simulink model "fft32kpt_ssr16_fixed"  (R2024b)
settings: Solver=VariableStepAuto  StartTime=0.0  StopTime=sample_period*N*5  RelTol=1e-3
PreLoadFcn:
  | clk_freq = 570e6; % PL clock frequency
  | sample_period = 1/(570e6*16); % 570Msps*16parallel paths
  | N=32768; % fft point size
  | binw=(1/sample_period) / 2*N; % bin width
  | 
  | bin_freq = 2*pi*11*binw+pi*binw; % sin, cos freq centering per channel
  | 
  | % for transpose block
  | DATA_WIDTH=16;
  | SSR=16;
  | M=16;
  | N1=N/M;
  | MEM_STYLE=4; % MEM OPTIONS: 4 - ULTRA, 0 - AUTO, 1 - BRAM, 5 - MIXED
InitFcn:
  | clk_freq = 570e6; % PL clock frequency
  | sample_period = 1/(570e6*16); % 570Msps*16parallel paths
  | N=32768; % fft point size
  | binw=(1/sample_period) / 2*N; % bin width
  | 
  | bin_freq = 2*pi*11*binw+pi*binw; % sin, cos freq centering per channel
  | 
  | % for transpose block
  | DATA_WIDTH=16;
  | SSR=16;
  | M=16;
  | N1=N/M;
  | MEM_STYLE=4; % MEM OPTIONS: 4 - ULTRA, 0 - AUTO, 1 - BRAM, 5 - MIXED
undefined symbols (not defined in the file or in its folder): None, S, vsva2197, xcvc1902
libraries: aieBasic x47, hdlBasic x39, aieUtilities x16, aieDSP x16, hdlUtilities x16, matrix_library x16, hdlSSR x13, simulink x1, dspxfrm3 x1, vmcUtilities x1
(part 2 of 3)

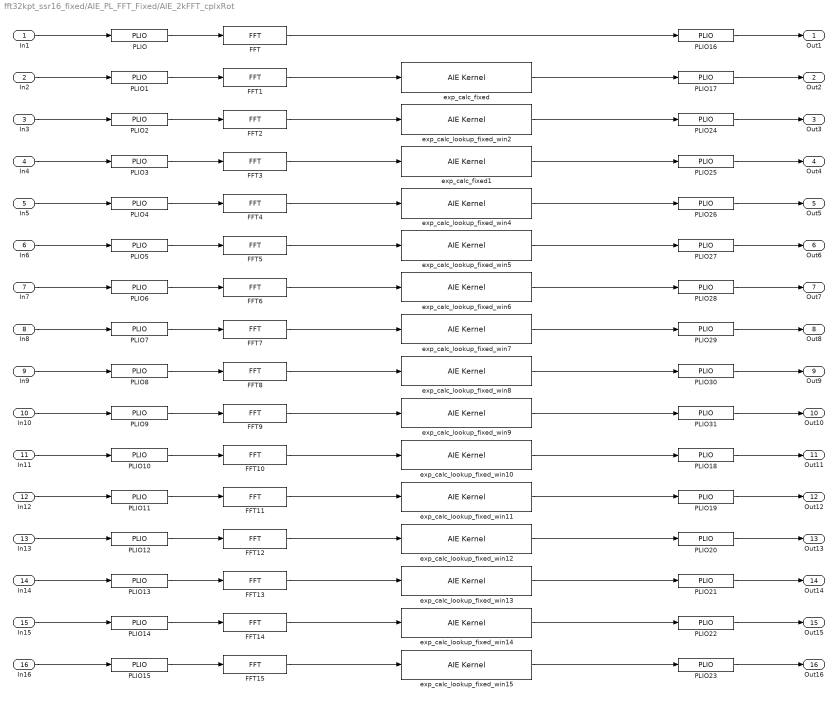
== system fft32kpt_ssr16_fixed/AIE_PL_FFT_Fixed/AIE_2kFFT_cplxRot ==
  In1 : Inport
  In2 : Inport  Port=2
  In3 : Inport  Port=3
  In4 : Inport  Port=4
  In5 : Inport  Port=5
  In6 : Inport  Port=6
  In7 : Inport  Port=7
  In8 : Inport  Port=8
  In9 : Inport  Port=9
  In10 : Inport  Port=10
  In11 : Inport  Port=11
  In12 : Inport  Port=12
  In13 : Inport  Port=13
  In14 : Inport  Port=14
  In15 : Inport  Port=15
  In16 : Inport  Port=16
  FFT{,1..15} (16 alike) : aieDSP/FFT  AIE_VARIANT=1  data_type=cint16  data_out_type=cint16  twiddle_type=cint16  point_size=2048  input_window_size=2048  shift_val=11  rnd_mode=Round symmetrical to infinity  sat_mode=0-None  ssr=1  twiddle_mode=0  use_ssr_widget_kernels=off  casc_length=1  transform_fft_nifft=1  TP_API=0  TP_DYN_PT_SIZE=0  blockJsonConstraints=[]  blockJsonConstraintsInternal=[]  spec=vmc_fft.json  SerializedMaskParamNames=[]  SerializedMaskParamValues=[]  SerializedMaskParamVisibilities=[]  block_type=FFT  SerializedMaskParamDataypes=uint|typename|typename|typename|uint|uint|uint|uint|uint|uint|uint|uint|uint|uint|uint|uint  SerializedMaskParamEnumStrArr=0|0|0|0|0|0|0|Round to positive infinity,Round to negative infinity,Round symmetrical to infinity,Round symmetrical to zero,Round convergent to even,Round convergent to odd|0-None,1-Asymmetric,3-Symmetric|0|0|0|0|0|0|0  SerializedMaskParamEnumValArr=0|0|0|0|0|0|0|2,3,4,5,6,7|0,1,3|0|0|0|0|0|0|0  SerializedMaskParamVectorArr=0|0|0|0|0|0|0|0|0|0|0|0|0|0|0|0  SerializedMaskParamKeys=AIE_VARIANT|TT_DATA|TT_OUT_DATA|TT_TWIDDLE|TP_POINT_SIZE|TP_WINDOW_VSIZE|TP_SHIFT|TP_RND|TP_SAT|TP_PARALLEL_POWER|TP_TWIDDLE_MODE|TP_USE_WIDGETS|TP_CASC_LEN|TP_FFT_NIFFT|TP_API|TP_DYN_PT_SIZE
  PLIO{,1..31} (32 alike) : aieBasic/PLIO  PlioWidth=64  PlioFreqSpec=on  PlioFreq=clk_freq/1e6  ColLocation=0  channel=0  blockJsonConstraints=[]  deprecateConstraints=0
  exp_calc_fixed : aieBasic/AIE Kernel  KernelAllAttrs=|  PortNames={'cb_input1'; 'cb_output1'}  PortSerializedTypes={'{Q2{R{Tadf::input_buffer{1{t{Scint16}}}}}}'; '{Q2{R{Tadf::output_buffer{1{t{Scint16}}}}}}'}  PortWindowSizes={2.048000000000000000e+03, 2.048000000000000000e+03}  PortWindowMargins={0.000000000000000000e+00, 0.000000000000000000e+00}  PortSynchronicities={'sync', 'sync'}  PortSignalSizes={0.000000000000000000e+00; 0.000000000000000000e+00}  FunctionTemplateSpecKind=implicit  FunctionTemplateParamNames={'PHASE_INDEX'}  FunctionTemplateParamKinds={'nontype'}  FunctionTemplateParamTypes={'unsigned int'}  FunctionTemplateParamValues={'1'}  FunctionIndex=1  FunctionTabVisible=on  FunctionTemplateParamsVisible=on  FunctionDeclTypeOptions=|  FunctionDecl=|  FunctionTemplateParams={ 'PHASE_INDEX', 'unsigned int', '1' }  FunctionTemplateParamsEnables={'off', 'off', 'on'}  PortAttrs={ 'input', 'cb_input1', 'adf::input_buffer< cint16 > & restrict', '2048', '0', 'sync', ''; 'output', 'cb_output1', 'adf::output_buffer< cint16 > & restrict', '2048', '', 'sync', '' }  PortAttrsEnables={'off', 'off', 'off', 'on', 'off', 'off', 'off';'off', 'off', 'off', 'on', 'off', 'off', 'off'}  SampleTime=-1  KernelHeaderFile=exp_calc_fixed.h  KernelFunction=exp_calc_fixed  KernelSourceFile=exp_calc_fixed.cc  KernelSearchPaths={}  PreProcOptions={}  blockJsonConstraints="{\"type\":\"constraint\",\"constraintType\":\"coreUtilization\",\"sid\":\"3274\",\"lhs\":{\"type\":\"runtimeRatio\",\"args\":{\"type\":\"kernel\",\"name\":\"fft32kpt_int_xpose_rrlto/AIE_2kFFT_cplxRot/exp_calc_lookup_fixed_win1\",\"sid\":\"3274\"}},\"rhs\":{\"type\":\"evaluable\",\"expr\":\"0.2\",\"value\":0.2},\"equality\":true}"
      KernelAllAttrs=|
      | s[12;12;9;9;19;14;21;23;21;23;24;21;15;17;12;24;26;26;26;27;28;9;21;23;23;23;24;25;14;19;19;29]@FunctionNameDeclFileNamePortNamesPortTypesPortSerializedTypesPortDirectionsPortWindowSizeEnablesPortWindowMarginEnablesPortBufferSizeEnablesPortBufferMarginEnablesPortSynchronicityEnablesPortSignalSizeEnablesPortBufferSizesPortBufferMarginsFunctionDeclFunctionTemplateSpecKindFunctionTemplateParamNamesFunctionTemplateParamKindsFunctionTemplateParamTypesFunctionTemplateParamValuesFunctionTemplateParamEnablesClassDeclClassTemplateSpecKindClassTemplateParamNamesClassTemplateParamKindsClassTemplateParamTypesClassTemplateParamValuesClassTemplateParamEnablesClassCtorDeclsClassCtorParamNamesClassCtorParamTypesClassCtorParamSerializedTypes[1 1]@C[32 1]@t14@exp_calc_fixedt22@../../exp_calc_fixed.hC[2 1]@t9@cb_input1t10@cb_output1C[2 1]@t38@adf::input_buffer< cint16 > & restrictt39@adf::output_buffer< cint16 > & restrictC[2 1]@t42@{Q2{R{Tadf::input_buffer{1{t{Scint16}}}}}}t43@{Q2{R{Tadf::output_buffer{1{t{Scint16}}}}}}C[2 1]@t5@inputt6@outputC[2 1]@l1@l1@C[2 1]@l1@l0@C[2 1]@l1@l1@C[2 1]@l0@l0@C[2 1]@l1@l1@C[2 1]@l0@l0@C[2 1]@nnC[2 1]@nnt160@template < unsigned int PHASE_INDEX > 
      | void exp_calc_fixed(adf::input_buffer< cint16 > & restrict cb_input1, adf::output_buffer< cint16 > & restrict cb_output1)t8@implicitC[1 1]@t11@PHASE_INDEXC[1 1]@t7@nontypeC[1 1]@t12@unsigned intC[1 1]@nC[1 1]@l1@nne[0 1]@e[0 1]@e[0 1]@e[0 1]@e[0 1]@e[0 1]@e[0 1]@e[0 1]@e[0 1]@
      FunctionDeclTypeOptions=|
      | C[1 1]@t162@template < unsigned int PHASE_INDEX > 
      | void exp_calc_fixed(adf::input_buffer< cint16 > && restrict cb_input1, adf::output_buffer< cint16 > && restrict cb_output1)
      FunctionDecl=|
      | template < unsigned int PHASE_INDEX > 
      | void exp_calc_fixed(adf::input_buffer< cint16 > && restrict cb_input1, adf::output_buffer< cint16 > && restrict cb_output1)
  exp_calc_fixed1 : aieBasic/AIE Kernel  KernelAllAttrs=|  PortNames={'cb_input1'; 'cb_output1'}  PortSerializedTypes={'{Q2{R{Tadf::input_buffer{1{t{Scint16}}}}}}'; '{Q2{R{Tadf::output_buffer{1{t{Scint16}}}}}}'}  PortWindowSizes={2.048000000000000000e+03, 2.048000000000000000e+03}  PortWindowMargins={0.000000000000000000e+00, 0.000000000000000000e+00}  PortSynchronicities={'sync', 'sync'}  PortSignalSizes={0.000000000000000000e+00; 0.000000000000000000e+00}  FunctionTemplateSpecKind=implicit  FunctionTemplateParamNames={'PHASE_INDEX'}  FunctionTemplateParamKinds={'nontype'}  FunctionTemplateParamTypes={'unsigned int'}  FunctionTemplateParamValues={'3'}  FunctionIndex=1  FunctionTabVisible=on  FunctionTemplateParamsVisible=on  FunctionDeclTypeOptions=|  FunctionDecl=|  FunctionTemplateParams={ 'PHASE_INDEX', 'unsigned int', '3' }  FunctionTemplateParamsEnables={'off', 'off', 'on'}  PortAttrs={ 'input', 'cb_input1', 'adf::input_buffer< cint16 > & restrict', '2048', '0', 'sync', ''; 'output', 'cb_output1', 'adf::output_buffer< cint16 > & restrict', '2048', '', 'sync', '' }  PortAttrsEnables={'off', 'off', 'off', 'on', 'off', 'off', 'off';'off', 'off', 'off', 'on', 'off', 'off', 'off'}  SampleTime=-1  KernelHeaderFile=exp_calc_fixed.h  KernelFunction=exp_calc_fixed  KernelSourceFile=exp_calc_fixed.cc  KernelSearchPaths={}  PreProcOptions={}  blockJsonConstraints="{\"type\":\"constraint\",\"constraintType\":\"coreUtilization\",\"sid\":\"3282\",\"lhs\":{\"type\":\"runtimeRatio\",\"args\":{\"type\":\"kernel\",\"name\":\"fft32kpt_int_xpose/AIE_2kFFT_cplxRot/exp_calc_lookup_fixed_win3\",\"sid\":\"3282\"}},\"rhs\":{\"type\":\"evaluable\",\"expr\":\"0.2\",\"value\":0.2},\"equality\":true}"
      KernelAllAttrs=|
      | s[12;12;9;9;19;14;21;23;21;23;24;21;15;17;12;24;26;26;26;27;28;9;21;23;23;23;24;25;14;19;19;29]@FunctionNameDeclFileNamePortNamesPortTypesPortSerializedTypesPortDirectionsPortWindowSizeEnablesPortWindowMarginEnablesPortBufferSizeEnablesPortBufferMarginEnablesPortSynchronicityEnablesPortSignalSizeEnablesPortBufferSizesPortBufferMarginsFunctionDeclFunctionTemplateSpecKindFunctionTemplateParamNamesFunctionTemplateParamKindsFunctionTemplateParamTypesFunctionTemplateParamValuesFunctionTemplateParamEnablesClassDeclClassTemplateSpecKindClassTemplateParamNamesClassTemplateParamKindsClassTemplateParamTypesClassTemplateParamValuesClassTemplateParamEnablesClassCtorDeclsClassCtorParamNamesClassCtorParamTypesClassCtorParamSerializedTypes[1 1]@C[32 1]@t14@exp_calc_fixedt22@../../exp_calc_fixed.hC[2 1]@t9@cb_input1t10@cb_output1C[2 1]@t38@adf::input_buffer< cint16 > & restrictt39@adf::output_buffer< cint16 > & restrictC[2 1]@t42@{Q2{R{Tadf::input_buffer{1{t{Scint16}}}}}}t43@{Q2{R{Tadf::output_buffer{1{t{Scint16}}}}}}C[2 1]@t5@inputt6@outputC[2 1]@l1@l1@C[2 1]@l1@l0@C[2 1]@l1@l1@C[2 1]@l0@l0@C[2 1]@l1@l1@C[2 1]@l0@l0@C[2 1]@nnC[2 1]@nnt160@template < unsigned int PHASE_INDEX > 
      | void exp_calc_fixed(adf::input_buffer< cint16 > & restrict cb_input1, adf::output_buffer< cint16 > & restrict cb_output1)t8@implicitC[1 1]@t11@PHASE_INDEXC[1 1]@t7@nontypeC[1 1]@t12@unsigned intC[1 1]@nC[1 1]@l1@nne[0 1]@e[0 1]@e[0 1]@e[0 1]@e[0 1]@e[0 1]@e[0 1]@e[0 1]@e[0 1]@
      FunctionDeclTypeOptions=|
      | C[1 1]@t162@template < unsigned int PHASE_INDEX > 
      | void exp_calc_fixed(adf::input_buffer< cint16 > && restrict cb_input1, adf::output_buffer< cint16 > && restrict cb_output1)
      FunctionDecl=|
      | template < unsigned int PHASE_INDEX > 
      | void exp_calc_fixed(adf::input_buffer< cint16 > && restrict cb_input1, adf::output_buffer< cint16 > && restrict cb_output1)
  exp_calc_lookup_fixed_win10 : aieBasic/AIE Kernel  KernelAllAttrs=|  PortNames={'cb_input1'; 'cb_output1'}  PortSerializedTypes={'{Q2{R{Tadf::input_buffer{1{t{Scint16}}}}}}'; '{Q2{R{Tadf::output_buffer{1{t{Scint16}}}}}}'}  PortWindowSizes={2.048000000000000000e+03, 2.048000000000000000e+03}  PortWindowMargins={0.000000000000000000e+00, 0.000000000000000000e+00}  PortSynchronicities={'sync', 'sync'}  PortSignalSizes={0.000000000000000000e+00; 0.000000000000000000e+00}  FunctionTemplateSpecKind=implicit  FunctionTemplateParamNames={'PHASE_INDEX'}  FunctionTemplateParamKinds={'nontype'}  FunctionTemplateParamTypes={'unsigned int'}  FunctionTemplateParamValues={'10'}  FunctionIndex=1  FunctionTabVisible=on  FunctionTemplateParamsVisible=on  FunctionDeclTypeOptions=|  FunctionDecl=|  FunctionTemplateParams={ 'PHASE_INDEX', 'unsigned int', '10' }  FunctionTemplateParamsEnables={'off', 'off', 'on'}  PortAttrs={ 'input', 'cb_input1', 'adf::input_buffer< cint16 > & restrict', '2048', '0', 'sync', ''; 'output', 'cb_output1', 'adf::output_buffer< cint16 > & restrict', '2048', '', 'sync', '' }  PortAttrsEnables={'off', 'off', 'off', 'on', 'off', 'off', 'off';'off', 'off', 'off', 'on', 'off', 'off', 'off'}  SampleTime=-1  KernelHeaderFile=exp_calc_fixed.h  KernelFunction=exp_calc_fixed  KernelSourceFile=exp_calc_fixed.cc  KernelSearchPaths={}  PreProcOptions={}  blockJsonConstraints="{\"type\":\"constraint\",\"constraintType\":\"coreUtilization\",\"sid\":\"3275\",\"lhs\":{\"type\":\"runtimeRatio\",\"args\":{\"type\":\"kernel\",\"name\":\"fft32kpt_int_xpose_rrlto/AIE_2kFFT_cplxRot/exp_calc_lookup_fixed_win10\",\"sid\":\"3275\"}},\"rhs\":{\"type\":\"evaluable\",\"expr\":\"0.2\",\"value\":0.2},\"equality\":true}"
      KernelAllAttrs=|
      | s[12;12;9;9;19;14;21;23;21;23;24;21;15;17;12;24;26;26;26;27;28;9;21;23;23;23;24;25;14;19;19;29]@FunctionNameDeclFileNamePortNamesPortTypesPortSerializedTypesPortDirectionsPortWindowSizeEnablesPortWindowMarginEnablesPortBufferSizeEnablesPortBufferMarginEnablesPortSynchronicityEnablesPortSignalSizeEnablesPortBufferSizesPortBufferMarginsFunctionDeclFunctionTemplateSpecKindFunctionTemplateParamNamesFunctionTemplateParamKindsFunctionTemplateParamTypesFunctionTemplateParamValuesFunctionTemplateParamEnablesClassDeclClassTemplateSpecKindClassTemplateParamNamesClassTemplateParamKindsClassTemplateParamTypesClassTemplateParamValuesClassTemplateParamEnablesClassCtorDeclsClassCtorParamNamesClassCtorParamTypesClassCtorParamSerializedTypes[1 1]@C[32 1]@t14@exp_calc_fixedt22@../../exp_calc_fixed.hC[2 1]@t9@cb_input1t10@cb_output1C[2 1]@t38@adf::input_buffer< cint16 > & restrictt39@adf::output_buffer< cint16 > & restrictC[2 1]@t42@{Q2{R{Tadf::input_buffer{1{t{Scint16}}}}}}t43@{Q2{R{Tadf::output_buffer{1{t{Scint16}}}}}}C[2 1]@t5@inputt6@outputC[2 1]@l1@l1@C[2 1]@l1@l0@C[2 1]@l1@l1@C[2 1]@l0@l0@C[2 1]@l1@l1@C[2 1]@l0@l0@C[2 1]@nnC[2 1]@nnt160@template < unsigned int PHASE_INDEX > 
      | void exp_calc_fixed(adf::input_buffer< cint16 > & restrict cb_input1, adf::output_buffer< cint16 > & restrict cb_output1)t8@implicitC[1 1]@t11@PHASE_INDEXC[1 1]@t7@nontypeC[1 1]@t12@unsigned intC[1 1]@nC[1 1]@l1@nne[0 1]@e[0 1]@e[0 1]@e[0 1]@e[0 1]@e[0 1]@e[0 1]@e[0 1]@e[0 1]@
      FunctionDeclTypeOptions=|
      | C[1 1]@t162@template < unsigned int PHASE_INDEX > 
      | void exp_calc_fixed(adf::input_buffer< cint16 > && restrict cb_input1, adf::output_buffer< cint16 > && restrict cb_output1)
      FunctionDecl=|
      | template < unsigned int PHASE_INDEX > 
      | void exp_calc_fixed(adf::input_buffer< cint16 > && restrict cb_input1, adf::output_buffer< cint16 > && restrict cb_output1)
  exp_calc_lookup_fixed_win11 : aieBasic/AIE Kernel  KernelAllAttrs=|  PortNames={'cb_input1'; 'cb_output1'}  PortSerializedTypes={'{Q2{R{Tadf::input_buffer{1{t{Scint16}}}}}}'; '{Q2{R{Tadf::output_buffer{1{t{Scint16}}}}}}'}  PortWindowSizes={2.048000000000000000e+03, 2.048000000000000000e+03}  PortWindowMargins={0.000000000000000000e+00, 0.000000000000000000e+00}  PortSynchronicities={'sync', 'sync'}  PortSignalSizes={0.000000000000000000e+00; 0.000000000000000000e+00}  FunctionTemplateSpecKind=implicit  FunctionTemplateParamNames={'PHASE_INDEX'}  FunctionTemplateParamKinds={'nontype'}  FunctionTemplateParamTypes={'unsigned int'}  FunctionTemplateParamValues={'11'}  FunctionIndex=1  FunctionTabVisible=on  FunctionTemplateParamsVisible=on  FunctionDeclTypeOptions=|  FunctionDecl=|  FunctionTemplateParams={ 'PHASE_INDEX', 'unsigned int', '11' }  FunctionTemplateParamsEnables={'off', 'off', 'on'}  PortAttrs={ 'input', 'cb_input1', 'adf::input_buffer< cint16 > & restrict', '2048', '0', 'sync', ''; 'output', 'cb_output1', 'adf::output_buffer< cint16 > & restrict', '2048', '', 'sync', '' }  PortAttrsEnables={'off', 'off', 'off', 'on', 'off', 'off', 'off';'off', 'off', 'off', 'on', 'off', 'off', 'off'}  SampleTime=-1  KernelHeaderFile=exp_calc_fixed.h  KernelFunction=exp_calc_fixed  KernelSourceFile=exp_calc_fixed.cc  KernelSearchPaths={}  PreProcOptions={}  blockJsonConstraints="{\"type\":\"constraint\",\"constraintType\":\"coreUtilization\",\"sid\":\"3276\",\"lhs\":{\"type\":\"runtimeRatio\",\"args\":{\"type\":\"kernel\",\"name\":\"fft32kpt_int_xpose/AIE_2kFFT_cplxRot/exp_calc_lookup_fixed_win11\",\"sid\":\"3276\"}},\"rhs\":{\"type\":\"evaluable\",\"expr\":\"0.2\",\"value\":0.2},\"equality\":true}"
      KernelAllAttrs=|
      | s[12;12;9;9;19;14;21;23;21;23;24;21;15;17;12;24;26;26;26;27;28;9;21;23;23;23;24;25;14;19;19;29]@FunctionNameDeclFileNamePortNamesPortTypesPortSerializedTypesPortDirectionsPortWindowSizeEnablesPortWindowMarginEnablesPortBufferSizeEnablesPortBufferMarginEnablesPortSynchronicityEnablesPortSignalSizeEnablesPortBufferSizesPortBufferMarginsFunctionDeclFunctionTemplateSpecKindFunctionTemplateParamNamesFunctionTemplateParamKindsFunctionTemplateParamTypesFunctionTemplateParamValuesFunctionTemplateParamEnablesClassDeclClassTemplateSpecKindClassTemplateParamNamesClassTemplateParamKindsClassTemplateParamTypesClassTemplateParamValuesClassTemplateParamEnablesClassCtorDeclsClassCtorParamNamesClassCtorParamTypesClassCtorParamSerializedTypes[1 1]@C[32 1]@t14@exp_calc_fixedt22@../../exp_calc_fixed.hC[2 1]@t9@cb_input1t10@cb_output1C[2 1]@t38@adf::input_buffer< cint16 > & restrictt39@adf::output_buffer< cint16 > & restrictC[2 1]@t42@{Q2{R{Tadf::input_buffer{1{t{Scint16}}}}}}t43@{Q2{R{Tadf::output_buffer{1{t{Scint16}}}}}}C[2 1]@t5@inputt6@outputC[2 1]@l1@l1@C[2 1]@l1@l0@C[2 1]@l1@l1@C[2 1]@l0@l0@C[2 1]@l1@l1@C[2 1]@l0@l0@C[2 1]@nnC[2 1]@nnt160@template < unsigned int PHASE_INDEX > 
      | void exp_calc_fixed(adf::input_buffer< cint16 > & restrict cb_input1, adf::output_buffer< cint16 > & restrict cb_output1)t8@implicitC[1 1]@t11@PHASE_INDEXC[1 1]@t7@nontypeC[1 1]@t12@unsigned intC[1 1]@nC[1 1]@l1@nne[0 1]@e[0 1]@e[0 1]@e[0 1]@e[0 1]@e[0 1]@e[0 1]@e[0 1]@e[0 1]@
      FunctionDeclTypeOptions=|
      | C[1 1]@t162@template < unsigned int PHASE_INDEX > 
      | void exp_calc_fixed(adf::input_buffer< cint16 > && restrict cb_input1, adf::output_buffer< cint16 > && restrict cb_output1)
      FunctionDecl=|
      | template < unsigned int PHASE_INDEX > 
      | void exp_calc_fixed(adf::input_buffer< cint16 > && restrict cb_input1, adf::output_buffer< cint16 > && restrict cb_output1)
  exp_calc_lookup_fixed_win12 : aieBasic/AIE Kernel  KernelAllAttrs=|  PortNames={'cb_input1'; 'cb_output1'}  PortSerializedTypes={'{Q2{R{Tadf::input_buffer{1{t{Scint16}}}}}}'; '{Q2{R{Tadf::output_buffer{1{t{Scint16}}}}}}'}  PortWindowSizes={2.048000000000000000e+03, 2.048000000000000000e+03}  PortWindowMargins={0.000000000000000000e+00, 0.000000000000000000e+00}  PortSynchronicities={'sync', 'sync'}  PortSignalSizes={0.000000000000000000e+00; 0.000000000000000000e+00}  FunctionTemplateSpecKind=implicit  FunctionTemplateParamNames={'PHASE_INDEX'}  FunctionTemplateParamKinds={'nontype'}  FunctionTemplateParamTypes={'unsigned int'}  FunctionTemplateParamValues={'12'}  FunctionIndex=1  FunctionTabVisible=on  FunctionTemplateParamsVisible=on  FunctionDeclTypeOptions=|  FunctionDecl=|  FunctionTemplateParams={ 'PHASE_INDEX', 'unsigned int', '12' }  FunctionTemplateParamsEnables={'off', 'off', 'on'}  PortAttrs={ 'input', 'cb_input1', 'adf::input_buffer< cint16 > & restrict', '2048', '0', 'sync', ''; 'output', 'cb_output1', 'adf::output_buffer< cint16 > & restrict', '2048', '', 'sync', '' }  PortAttrsEnables={'off', 'off', 'off', 'on', 'off', 'off', 'off';'off', 'off', 'off', 'on', 'off', 'off', 'off'}  SampleTime=-1  KernelHeaderFile=exp_calc_fixed.h  KernelFunction=exp_calc_fixed  KernelSourceFile=exp_calc_fixed.cc  KernelSearchPaths={}  PreProcOptions={}  blockJsonConstraints="{\"type\":\"constraint\",\"constraintType\":\"coreUtilization\",\"sid\":\"3277\",\"lhs\":{\"type\":\"runtimeRatio\",\"args\":{\"type\":\"kernel\",\"name\":\"fft32kpt_int_xpose/AIE_2kFFT_cplxRot/exp_calc_lookup_fixed_win12\",\"sid\":\"3277\"}},\"rhs\":{\"type\":\"evaluable\",\"expr\":\"0.2\",\"value\":0.2},\"equality\":true}"
      KernelAllAttrs=|
      | s[12;12;9;9;19;14;21;23;21;23;24;21;15;17;12;24;26;26;26;27;28;9;21;23;23;23;24;25;14;19;19;29]@FunctionNameDeclFileNamePortNamesPortTypesPortSerializedTypesPortDirectionsPortWindowSizeEnablesPortWindowMarginEnablesPortBufferSizeEnablesPortBufferMarginEnablesPortSynchronicityEnablesPortSignalSizeEnablesPortBufferSizesPortBufferMarginsFunctionDeclFunctionTemplateSpecKindFunctionTemplateParamNamesFunctionTemplateParamKindsFunctionTemplateParamTypesFunctionTemplateParamValuesFunctionTemplateParamEnablesClassDeclClassTemplateSpecKindClassTemplateParamNamesClassTemplateParamKindsClassTemplateParamTypesClassTemplateParamValuesClassTemplateParamEnablesClassCtorDeclsClassCtorParamNamesClassCtorParamTypesClassCtorParamSerializedTypes[1 1]@C[32 1]@t14@exp_calc_fixedt22@../../exp_calc_fixed.hC[2 1]@t9@cb_input1t10@cb_output1C[2 1]@t38@adf::input_buffer< cint16 > & restrictt39@adf::output_buffer< cint16 > & restrictC[2 1]@t42@{Q2{R{Tadf::input_buffer{1{t{Scint16}}}}}}t43@{Q2{R{Tadf::output_buffer{1{t{Scint16}}}}}}C[2 1]@t5@inputt6@outputC[2 1]@l1@l1@C[2 1]@l1@l0@C[2 1]@l1@l1@C[2 1]@l0@l0@C[2 1]@l1@l1@C[2 1]@l0@l0@C[2 1]@nnC[2 1]@nnt160@template < unsigned int PHASE_INDEX > 
      | void exp_calc_fixed(adf::input_buffer< cint16 > & restrict cb_input1, adf::output_buffer< cint16 > & restrict cb_output1)t8@implicitC[1 1]@t11@PHASE_INDEXC[1 1]@t7@nontypeC[1 1]@t12@unsigned intC[1 1]@nC[1 1]@l1@nne[0 1]@e[0 1]@e[0 1]@e[0 1]@e[0 1]@e[0 1]@e[0 1]@e[0 1]@e[0 1]@
      FunctionDeclTypeOptions=|
      | C[1 1]@t162@template < unsigned int PHASE_INDEX > 
      | void exp_calc_fixed(adf::input_buffer< cint16 > && restrict cb_input1, adf::output_buffer< cint16 > && restrict cb_output1)
      FunctionDecl=|
      | template < unsigned int PHASE_INDEX > 
      | void exp_calc_fixed(adf::input_buffer< cint16 > && restrict cb_input1, adf::output_buffer< cint16 > && restrict cb_output1)
  exp_calc_lookup_fixed_win13 : aieBasic/AIE Kernel  KernelAllAttrs=|  PortNames={'cb_input1'; 'cb_output1'}  PortSerializedTypes={'{Q2{R{Tadf::input_buffer{1{t{Scint16}}}}}}'; '{Q2{R{Tadf::output_buffer{1{t{Scint16}}}}}}'}  PortWindowSizes={2.048000000000000000e+03, 2.048000000000000000e+03}  PortWindowMargins={0.000000000000000000e+00, 0.000000000000000000e+00}  PortSynchronicities={'sync', 'sync'}  PortSignalSizes={0.000000000000000000e+00; 0.000000000000000000e+00}  FunctionTemplateSpecKind=implicit  FunctionTemplateParamNames={'PHASE_INDEX'}  FunctionTemplateParamKinds={'nontype'}  FunctionTemplateParamTypes={'unsigned int'}  FunctionTemplateParamValues={'13'}  FunctionIndex=1  FunctionTabVisible=on  FunctionTemplateParamsVisible=on  FunctionDeclTypeOptions=|  FunctionDecl=|  FunctionTemplateParams={ 'PHASE_INDEX', 'unsigned int', '13' }  FunctionTemplateParamsEnables={'off', 'off', 'on'}  PortAttrs={ 'input', 'cb_input1', 'adf::input_buffer< cint16 > & restrict', '2048', '0', 'sync', ''; 'output', 'cb_output1', 'adf::output_buffer< cint16 > & restrict', '2048', '', 'sync', '' }  PortAttrsEnables={'off', 'off', 'off', 'on', 'off', 'off', 'off';'off', 'off', 'off', 'on', 'off', 'off', 'off'}  SampleTime=-1  KernelHeaderFile=exp_calc_fixed.h  KernelFunction=exp_calc_fixed  KernelSourceFile=exp_calc_fixed.cc  KernelSearchPaths={}  PreProcOptions={}  blockJsonConstraints="{\"type\":\"constraint\",\"constraintType\":\"coreUtilization\",\"sid\":\"3278\",\"lhs\":{\"type\":\"runtimeRatio\",\"args\":{\"type\":\"kernel\",\"name\":\"fft32kpt_int_xpose/AIE_2kFFT_cplxRot/exp_calc_lookup_fixed_win13\",\"sid\":\"3278\"}},\"rhs\":{\"type\":\"evaluable\",\"expr\":\"0.2\",\"value\":0.2},\"equality\":true}"
      KernelAllAttrs=|
      | s[12;12;9;9;19;14;21;23;21;23;24;21;15;17;12;24;26;26;26;27;28;9;21;23;23;23;24;25;14;19;19;29]@FunctionNameDeclFileNamePortNamesPortTypesPortSerializedTypesPortDirectionsPortWindowSizeEnablesPortWindowMarginEnablesPortBufferSizeEnablesPortBufferMarginEnablesPortSynchronicityEnablesPortSignalSizeEnablesPortBufferSizesPortBufferMarginsFunctionDeclFunctionTemplateSpecKindFunctionTemplateParamNamesFunctionTemplateParamKindsFunctionTemplateParamTypesFunctionTemplateParamValuesFunctionTemplateParamEnablesClassDeclClassTemplateSpecKindClassTemplateParamNamesClassTemplateParamKindsClassTemplateParamTypesClassTemplateParamValuesClassTemplateParamEnablesClassCtorDeclsClassCtorParamNamesClassCtorParamTypesClassCtorParamSerializedTypes[1 1]@C[32 1]@t14@exp_calc_fixedt22@../../exp_calc_fixed.hC[2 1]@t9@cb_input1t10@cb_output1C[2 1]@t38@adf::input_buffer< cint16 > & restrictt39@adf::output_buffer< cint16 > & restrictC[2 1]@t42@{Q2{R{Tadf::input_buffer{1{t{Scint16}}}}}}t43@{Q2{R{Tadf::output_buffer{1{t{Scint16}}}}}}C[2 1]@t5@inputt6@outputC[2 1]@l1@l1@C[2 1]@l1@l0@C[2 1]@l1@l1@C[2 1]@l0@l0@C[2 1]@l1@l1@C[2 1]@l0@l0@C[2 1]@nnC[2 1]@nnt160@template < unsigned int PHASE_INDEX > 
      | void exp_calc_fixed(adf::input_buffer< cint16 > & restrict cb_input1, adf::output_buffer< cint16 > & restrict cb_output1)t8@implicitC[1 1]@t11@PHASE_INDEXC[1 1]@t7@nontypeC[1 1]@t12@unsigned intC[1 1]@nC[1 1]@l1@nne[0 1]@e[0 1]@e[0 1]@e[0 1]@e[0 1]@e[0 1]@e[0 1]@e[0 1]@e[0 1]@
      FunctionDeclTypeOptions=|
      | C[1 1]@t162@template < unsigned int PHASE_INDEX > 
      | void exp_calc_fixed(adf::input_buffer< cint16 > && restrict cb_input1, adf::output_buffer< cint16 > && restrict cb_output1)
      FunctionDecl=|
      | template < unsigned int PHASE_INDEX > 
      | void exp_calc_fixed(adf::input_buffer< cint16 > && restrict cb_input1, adf::output_buffer< cint16 > && restrict cb_output1)
  exp_calc_lookup_fixed_win14 : aieBasic/AIE Kernel  KernelAllAttrs=|  PortNames={'cb_input1'; 'cb_output1'}  PortSerializedTypes={'{Q2{R{Tadf::input_buffer{1{t{Scint16}}}}}}'; '{Q2{R{Tadf::output_buffer{1{t{Scint16}}}}}}'}  PortWindowSizes={2.048000000000000000e+03, 2.048000000000000000e+03}  PortWindowMargins={0.000000000000000000e+00, 0.000000000000000000e+00}  PortSynchronicities={'sync', 'sync'}  PortSignalSizes={0.000000000000000000e+00; 0.000000000000000000e+00}  FunctionTemplateSpecKind=implicit  FunctionTemplateParamNames={'PHASE_INDEX'}  FunctionTemplateParamKinds={'nontype'}  FunctionTemplateParamTypes={'unsigned int'}  FunctionTemplateParamValues={'14'}  FunctionIndex=1  FunctionTabVisible=on  FunctionTemplateParamsVisible=on  FunctionDeclTypeOptions=|  FunctionDecl=|  FunctionTemplateParams={ 'PHASE_INDEX', 'unsigned int', '14' }  FunctionTemplateParamsEnables={'off', 'off', 'on'}  PortAttrs={ 'input', 'cb_input1', 'adf::input_buffer< cint16 > & restrict', '2048', '0', 'sync', ''; 'output', 'cb_output1', 'adf::output_buffer< cint16 > & restrict', '2048', '', 'sync', '' }  PortAttrsEnables={'off', 'off', 'off', 'on', 'off', 'off', 'off';'off', 'off', 'off', 'on', 'off', 'off', 'off'}  SampleTime=-1  KernelHeaderFile=exp_calc_fixed.h  KernelFunction=exp_calc_fixed  KernelSourceFile=exp_calc_fixed.cc  KernelSearchPaths={}  PreProcOptions={}  blockJsonConstraints="{\"type\":\"constraint\",\"constraintType\":\"coreUtilization\",\"sid\":\"3279\",\"lhs\":{\"type\":\"runtimeRatio\",\"args\":{\"type\":\"kernel\",\"name\":\"fft32kpt_int_xpose/AIE_2kFFT_cplxRot/exp_calc_lookup_fixed_win14\",\"sid\":\"3279\"}},\"rhs\":{\"type\":\"evaluable\",\"expr\":\"0.2\",\"value\":0.2},\"equality\":true}"
      KernelAllAttrs=|
      | s[12;12;9;9;19;14;21;23;21;23;24;21;15;17;12;24;26;26;26;27;28;9;21;23;23;23;24;25;14;19;19;29]@FunctionNameDeclFileNamePortNamesPortTypesPortSerializedTypesPortDirectionsPortWindowSizeEnablesPortWindowMarginEnablesPortBufferSizeEnablesPortBufferMarginEnablesPortSynchronicityEnablesPortSignalSizeEnablesPortBufferSizesPortBufferMarginsFunctionDeclFunctionTemplateSpecKindFunctionTemplateParamNamesFunctionTemplateParamKindsFunctionTemplateParamTypesFunctionTemplateParamValuesFunctionTemplateParamEnablesClassDeclClassTemplateSpecKindClassTemplateParamNamesClassTemplateParamKindsClassTemplateParamTypesClassTemplateParamValuesClassTemplateParamEnablesClassCtorDeclsClassCtorParamNamesClassCtorParamTypesClassCtorParamSerializedTypes[1 1]@C[32 1]@t14@exp_calc_fixedt22@../../exp_calc_fixed.hC[2 1]@t9@cb_input1t10@cb_output1C[2 1]@t38@adf::input_buffer< cint16 > & restrictt39@adf::output_buffer< cint16 > & restrictC[2 1]@t42@{Q2{R{Tadf::input_buffer{1{t{Scint16}}}}}}t43@{Q2{R{Tadf::output_buffer{1{t{Scint16}}}}}}C[2 1]@t5@inputt6@outputC[2 1]@l1@l1@C[2 1]@l1@l0@C[2 1]@l1@l1@C[2 1]@l0@l0@C[2 1]@l1@l1@C[2 1]@l0@l0@C[2 1]@nnC[2 1]@nnt160@template < unsigned int PHASE_INDEX > 
      | void exp_calc_fixed(adf::input_buffer< cint16 > & restrict cb_input1, adf::output_buffer< cint16 > & restrict cb_output1)t8@implicitC[1 1]@t11@PHASE_INDEXC[1 1]@t7@nontypeC[1 1]@t12@unsigned intC[1 1]@nC[1 1]@l1@nne[0 1]@e[0 1]@e[0 1]@e[0 1]@e[0 1]@e[0 1]@e[0 1]@e[0 1]@e[0 1]@
      FunctionDeclTypeOptions=|
      | C[1 1]@t162@template < unsigned int PHASE_INDEX > 
      | void exp_calc_fixed(adf::input_buffer< cint16 > && restrict cb_input1, adf::output_buffer< cint16 > && restrict cb_output1)
      FunctionDecl=|
      | template < unsigned int PHASE_INDEX > 
      | void exp_calc_fixed(adf::input_buffer< cint16 > && restrict cb_input1, adf::output_buffer< cint16 > && restrict cb_output1)
  exp_calc_lookup_fixed_win15 : aieBasic/AIE Kernel  KernelAllAttrs=|  PortNames={'cb_input1'; 'cb_output1'}  PortSerializedTypes={'{Q2{R{Tadf::input_buffer{1{t{Scint16}}}}}}'; '{Q2{R{Tadf::output_buffer{1{t{Scint16}}}}}}'}  PortWindowSizes={2.048000000000000000e+03, 2.048000000000000000e+03}  PortWindowMargins={0.000000000000000000e+00, 0.000000000000000000e+00}  PortSynchronicities={'sync', 'sync'}  PortSignalSizes={0.000000000000000000e+00; 0.000000000000000000e+00}  FunctionTemplateSpecKind=implicit  FunctionTemplateParamNames={'PHASE_INDEX'}  FunctionTemplateParamKinds={'nontype'}  FunctionTemplateParamTypes={'unsigned int'}  FunctionTemplateParamValues={'15'}  FunctionIndex=1  FunctionTabVisible=on  FunctionTemplateParamsVisible=on  FunctionDeclTypeOptions=|  FunctionDecl=|  FunctionTemplateParams={ 'PHASE_INDEX', 'unsigned int', '15' }  FunctionTemplateParamsEnables={'off', 'off', 'on'}  PortAttrs={ 'input', 'cb_input1', 'adf::input_buffer< cint16 > & restrict', '2048', '0', 'sync', ''; 'output', 'cb_output1', 'adf::output_buffer< cint16 > & restrict', '2048', '', 'sync', '' }  PortAttrsEnables={'off', 'off', 'off', 'on', 'off', 'off', 'off';'off', 'off', 'off', 'on', 'off', 'off', 'off'}  SampleTime=-1  KernelHeaderFile=exp_calc_fixed.h  KernelFunction=exp_calc_fixed  KernelSourceFile=exp_calc_fixed.cc  KernelSearchPaths={}  PreProcOptions={}  blockJsonConstraints="{\"type\":\"constraint\",\"constraintType\":\"coreUtilization\",\"sid\":\"3280\",\"lhs\":{\"type\":\"runtimeRatio\",\"args\":{\"type\":\"kernel\",\"name\":\"fft32kpt_int_xpose/AIE_2kFFT_cplxRot/exp_calc_lookup_fixed_win15\",\"sid\":\"3280\"}},\"rhs\":{\"type\":\"evaluable\",\"expr\":\"0.2\",\"value\":0.2},\"equality\":true}"
      KernelAllAttrs=|
      | s[12;12;9;9;19;14;21;23;21;23;24;21;15;17;12;24;26;26;26;27;28;9;21;23;23;23;24;25;14;19;19;29]@FunctionNameDeclFileNamePortNamesPortTypesPortSerializedTypesPortDirectionsPortWindowSizeEnablesPortWindowMarginEnablesPortBufferSizeEnablesPortBufferMarginEnablesPortSynchronicityEnablesPortSignalSizeEnablesPortBufferSizesPortBufferMarginsFunctionDeclFunctionTemplateSpecKindFunctionTemplateParamNamesFunctionTemplateParamKindsFunctionTemplateParamTypesFunctionTemplateParamValuesFunctionTemplateParamEnablesClassDeclClassTemplateSpecKindClassTemplateParamNamesClassTemplateParamKindsClassTemplateParamTypesClassTemplateParamValuesClassTemplateParamEnablesClassCtorDeclsClassCtorParamNamesClassCtorParamTypesClassCtorParamSerializedTypes[1 1]@C[32 1]@t14@exp_calc_fixedt22@../../exp_calc_fixed.hC[2 1]@t9@cb_input1t10@cb_output1C[2 1]@t38@adf::input_buffer< cint16 > & restrictt39@adf::output_buffer< cint16 > & restrictC[2 1]@t42@{Q2{R{Tadf::input_buffer{1{t{Scint16}}}}}}t43@{Q2{R{Tadf::output_buffer{1{t{Scint16}}}}}}C[2 1]@t5@inputt6@outputC[2 1]@l1@l1@C[2 1]@l1@l0@C[2 1]@l1@l1@C[2 1]@l0@l0@C[2 1]@l1@l1@C[2 1]@l0@l0@C[2 1]@nnC[2 1]@nnt160@template < unsigned int PHASE_INDEX > 
      | void exp_calc_fixed(adf::input_buffer< cint16 > & restrict cb_input1, adf::output_buffer< cint16 > & restrict cb_output1)t8@implicitC[1 1]@t11@PHASE_INDEXC[1 1]@t7@nontypeC[1 1]@t12@unsigned intC[1 1]@nC[1 1]@l1@nne[0 1]@e[0 1]@e[0 1]@e[0 1]@e[0 1]@e[0 1]@e[0 1]@e[0 1]@e[0 1]@
      FunctionDeclTypeOptions=|
      | C[1 1]@t162@template < unsigned int PHASE_INDEX > 
      | void exp_calc_fixed(adf::input_buffer< cint16 > && restrict cb_input1, adf::output_buffer< cint16 > && restrict cb_output1)
      FunctionDecl=|
      | template < unsigned int PHASE_INDEX > 
      | void exp_calc_fixed(adf::input_buffer< cint16 > && restrict cb_input1, adf::output_buffer< cint16 > && restrict cb_output1)
  exp_calc_lookup_fixed_win2 : aieBasic/AIE Kernel  KernelAllAttrs=|  PortNames={'cb_input1'; 'cb_output1'}  PortSerializedTypes={'{Q2{R{Tadf::input_buffer{1{t{Scint16}}}}}}'; '{Q2{R{Tadf::output_buffer{1{t{Scint16}}}}}}'}  PortWindowSizes={2.048000000000000000e+03, 2.048000000000000000e+03}  PortWindowMargins={0.000000000000000000e+00, 0.000000000000000000e+00}  PortSynchronicities={'sync', 'sync'}  PortSignalSizes={0.000000000000000000e+00; 0.000000000000000000e+00}  FunctionTemplateSpecKind=implicit  FunctionTemplateParamNames={'PHASE_INDEX'}  FunctionTemplateParamKinds={'nontype'}  FunctionTemplateParamTypes={'unsigned int'}  FunctionTemplateParamValues={'2'}  FunctionIndex=1  FunctionTabVisible=on  FunctionTemplateParamsVisible=on  FunctionDeclTypeOptions=|  FunctionDecl=|  FunctionTemplateParams={ 'PHASE_INDEX', 'unsigned int', '2' }  FunctionTemplateParamsEnables={'off', 'off', 'on'}  PortAttrs={ 'input', 'cb_input1', 'adf::input_buffer< cint16 > & restrict', '2048', '0', 'sync', ''; 'output', 'cb_output1', 'adf::output_buffer< cint16 > & restrict', '2048', '', 'sync', '' }  PortAttrsEnables={'off', 'off', 'off', 'on', 'off', 'off', 'off';'off', 'off', 'off', 'on', 'off', 'off', 'off'}  SampleTime=-1  KernelHeaderFile=exp_calc_fixed.h  KernelFunction=exp_calc_fixed  KernelSourceFile=exp_calc_fixed.cc  KernelSearchPaths={}  PreProcOptions={}  blockJsonConstraints="{\"type\":\"constraint\",\"constraintType\":\"coreUtilization\",\"sid\":\"3281\",\"lhs\":{\"type\":\"runtimeRatio\",\"args\":{\"type\":\"kernel\",\"name\":\"fft32kpt_int_xpose/AIE_2kFFT_cplxRot/exp_calc_lookup_fixed_win2\",\"sid\":\"3281\"}},\"rhs\":{\"type\":\"evaluable\",\"expr\":\"0.2\",\"value\":0.2},\"equality\":true}"
      KernelAllAttrs=|
      | s[12;12;9;9;19;14;21;23;21;23;24;21;15;17;12;24;26;26;26;27;28;9;21;23;23;23;24;25;14;19;19;29]@FunctionNameDeclFileNamePortNamesPortTypesPortSerializedTypesPortDirectionsPortWindowSizeEnablesPortWindowMarginEnablesPortBufferSizeEnablesPortBufferMarginEnablesPortSynchronicityEnablesPortSignalSizeEnablesPortBufferSizesPortBufferMarginsFunctionDeclFunctionTemplateSpecKindFunctionTemplateParamNamesFunctionTemplateParamKindsFunctionTemplateParamTypesFunctionTemplateParamValuesFunctionTemplateParamEnablesClassDeclClassTemplateSpecKindClassTemplateParamNamesClassTemplateParamKindsClassTemplateParamTypesClassTemplateParamValuesClassTemplateParamEnablesClassCtorDeclsClassCtorParamNamesClassCtorParamTypesClassCtorParamSerializedTypes[1 1]@C[32 1]@t14@exp_calc_fixedt22@../../exp_calc_fixed.hC[2 1]@t9@cb_input1t10@cb_output1C[2 1]@t38@adf::input_buffer< cint16 > & restrictt39@adf::output_buffer< cint16 > & restrictC[2 1]@t42@{Q2{R{Tadf::input_buffer{1{t{Scint16}}}}}}t43@{Q2{R{Tadf::output_buffer{1{t{Scint16}}}}}}C[2 1]@t5@inputt6@outputC[2 1]@l1@l1@C[2 1]@l1@l0@C[2 1]@l1@l1@C[2 1]@l0@l0@C[2 1]@l1@l1@C[2 1]@l0@l0@C[2 1]@nnC[2 1]@nnt160@template < unsigned int PHASE_INDEX > 
      | void exp_calc_fixed(adf::input_buffer< cint16 > & restrict cb_input1, adf::output_buffer< cint16 > & restrict cb_output1)t8@implicitC[1 1]@t11@PHASE_INDEXC[1 1]@t7@nontypeC[1 1]@t12@unsigned intC[1 1]@nC[1 1]@l1@nne[0 1]@e[0 1]@e[0 1]@e[0 1]@e[0 1]@e[0 1]@e[0 1]@e[0 1]@e[0 1]@
      FunctionDeclTypeOptions=|
      | C[1 1]@t162@template < unsigned int PHASE_INDEX > 
      | void exp_calc_fixed(adf::input_buffer< cint16 > && restrict cb_input1, adf::output_buffer< cint16 > && restrict cb_output1)
      FunctionDecl=|
      | template < unsigned int PHASE_INDEX > 
      | void exp_calc_fixed(adf::input_buffer< cint16 > && restrict cb_input1, adf::output_buffer< cint16 > && restrict cb_output1)
  exp_calc_lookup_fixed_win4 : aieBasic/AIE Kernel  KernelAllAttrs=|  PortNames={'cb_input1'; 'cb_output1'}  PortSerializedTypes={'{Q2{R{Tadf::input_buffer{1{t{Scint16}}}}}}'; '{Q2{R{Tadf::output_buffer{1{t{Scint16}}}}}}'}  PortWindowSizes={2.048000000000000000e+03, 2.048000000000000000e+03}  PortWindowMargins={0.000000000000000000e+00, 0.000000000000000000e+00}  PortSynchronicities={'sync', 'sync'}  PortSignalSizes={0.000000000000000000e+00; 0.000000000000000000e+00}  FunctionTemplateSpecKind=implicit  FunctionTemplateParamNames={'PHASE_INDEX'}  FunctionTemplateParamKinds={'nontype'}  FunctionTemplateParamTypes={'unsigned int'}  FunctionTemplateParamValues={'4'}  FunctionIndex=1  FunctionTabVisible=on  FunctionTemplateParamsVisible=on  FunctionDeclTypeOptions=|  FunctionDecl=|  FunctionTemplateParams={ 'PHASE_INDEX', 'unsigned int', '4' }  FunctionTemplateParamsEnables={'off', 'off', 'on'}  PortAttrs={ 'input', 'cb_input1', 'adf::input_buffer< cint16 > & restrict', '2048', '0', 'sync', ''; 'output', 'cb_output1', 'adf::output_buffer< cint16 > & restrict', '2048', '', 'sync', '' }  PortAttrsEnables={'off', 'off', 'off', 'on', 'off', 'off', 'off';'off', 'off', 'off', 'on', 'off', 'off', 'off'}  SampleTime=-1  KernelHeaderFile=exp_calc_fixed.h  KernelFunction=exp_calc_fixed  KernelSourceFile=exp_calc_fixed.cc  KernelSearchPaths={}  PreProcOptions={}  blockJsonConstraints="{\"type\":\"constraint\",\"constraintType\":\"coreUtilization\",\"sid\":\"3283\",\"lhs\":{\"type\":\"runtimeRatio\",\"args\":{\"type\":\"kernel\",\"name\":\"fft32kpt_int_xpose/AIE_2kFFT_cplxRot/exp_calc_lookup_fixed_win4\",\"sid\":\"3283\"}},\"rhs\":{\"type\":\"evaluable\",\"expr\":\"0.2\",\"value\":0.2},\"equality\":true}"
      KernelAllAttrs=|
      | s[12;12;9;9;19;14;21;23;21;23;24;21;15;17;12;24;26;26;26;27;28;9;21;23;23;23;24;25;14;19;19;29]@FunctionNameDeclFileNamePortNamesPortTypesPortSerializedTypesPortDirectionsPortWindowSizeEnablesPortWindowMarginEnablesPortBufferSizeEnablesPortBufferMarginEnablesPortSynchronicityEnablesPortSignalSizeEnablesPortBufferSizesPortBufferMarginsFunctionDeclFunctionTemplateSpecKindFunctionTemplateParamNamesFunctionTemplateParamKindsFunctionTemplateParamTypesFunctionTemplateParamValuesFunctionTemplateParamEnablesClassDeclClassTemplateSpecKindClassTemplateParamNamesClassTemplateParamKindsClassTemplateParamTypesClassTemplateParamValuesClassTemplateParamEnablesClassCtorDeclsClassCtorParamNamesClassCtorParamTypesClassCtorParamSerializedTypes[1 1]@C[32 1]@t14@exp_calc_fixedt22@../../exp_calc_fixed.hC[2 1]@t9@cb_input1t10@cb_output1C[2 1]@t38@adf::input_buffer< cint16 > & restrictt39@adf::output_buffer< cint16 > & restrictC[2 1]@t42@{Q2{R{Tadf::input_buffer{1{t{Scint16}}}}}}t43@{Q2{R{Tadf::output_buffer{1{t{Scint16}}}}}}C[2 1]@t5@inputt6@outputC[2 1]@l1@l1@C[2 1]@l1@l0@C[2 1]@l1@l1@C[2 1]@l0@l0@C[2 1]@l1@l1@C[2 1]@l0@l0@C[2 1]@nnC[2 1]@nnt160@template < unsigned int PHASE_INDEX > 
      | void exp_calc_fixed(adf::input_buffer< cint16 > & restrict cb_input1, adf::output_buffer< cint16 > & restrict cb_output1)t8@implicitC[1 1]@t11@PHASE_INDEXC[1 1]@t7@nontypeC[1 1]@t12@unsigned intC[1 1]@nC[1 1]@l1@nne[0 1]@e[0 1]@e[0 1]@e[0 1]@e[0 1]@e[0 1]@e[0 1]@e[0 1]@e[0 1]@
      FunctionDeclTypeOptions=|
      | C[1 1]@t162@template < unsigned int PHASE_INDEX > 
      | void exp_calc_fixed(adf::input_buffer< cint16 > && restrict cb_input1, adf::output_buffer< cint16 > && restrict cb_output1)
      FunctionDecl=|
      | template < unsigned int PHASE_INDEX > 
      | void exp_calc_fixed(adf::input_buffer< cint16 > && restrict cb_input1, adf::output_buffer< cint16 > && restrict cb_output1)
  exp_calc_lookup_fixed_win5 : aieBasic/AIE Kernel  KernelAllAttrs=|  PortNames={'cb_input1'; 'cb_output1'}  PortSerializedTypes={'{Q2{R{Tadf::input_buffer{1{t{Scint16}}}}}}'; '{Q2{R{Tadf::output_buffer{1{t{Scint16}}}}}}'}  PortWindowSizes={2.048000000000000000e+03, 2.048000000000000000e+03}  PortWindowMargins={0.000000000000000000e+00, 0.000000000000000000e+00}  PortSynchronicities={'sync', 'sync'}  PortSignalSizes={0.000000000000000000e+00; 0.000000000000000000e+00}  FunctionTemplateSpecKind=implicit  FunctionTemplateParamNames={'PHASE_INDEX'}  FunctionTemplateParamKinds={'nontype'}  FunctionTemplateParamTypes={'unsigned int'}  FunctionTemplateParamValues={'5'}  FunctionIndex=1  FunctionTabVisible=on  FunctionTemplateParamsVisible=on  FunctionDeclTypeOptions=|  FunctionDecl=|  FunctionTemplateParams={ 'PHASE_INDEX', 'unsigned int', '5' }  FunctionTemplateParamsEnables={'off', 'off', 'on'}  PortAttrs={ 'input', 'cb_input1', 'adf::input_buffer< cint16 > & restrict', '2048', '0', 'sync', ''; 'output', 'cb_output1', 'adf::output_buffer< cint16 > & restrict', '2048', '', 'sync', '' }  PortAttrsEnables={'off', 'off', 'off', 'on', 'off', 'off', 'off';'off', 'off', 'off', 'on', 'off', 'off', 'off'}  SampleTime=-1  KernelHeaderFile=exp_calc_fixed.h  KernelFunction=exp_calc_fixed  KernelSourceFile=exp_calc_fixed.cc  KernelSearchPaths={}  PreProcOptions={}  blockJsonConstraints="{\"type\":\"constraint\",\"constraintType\":\"coreUtilization\",\"sid\":\"3284\",\"lhs\":{\"type\":\"runtimeRatio\",\"args\":{\"type\":\"kernel\",\"name\":\"fft32kpt_int_xpose/AIE_2kFFT_cplxRot/exp_calc_lookup_fixed_win5\",\"sid\":\"3284\"}},\"rhs\":{\"type\":\"evaluable\",\"expr\":\"0.2\",\"value\":0.2},\"equality\":true}"
      KernelAllAttrs=|
      | s[12;12;9;9;19;14;21;23;21;23;24;21;15;17;12;24;26;26;26;27;28;9;21;23;23;23;24;25;14;19;19;29]@FunctionNameDeclFileNamePortNamesPortTypesPortSerializedTypesPortDirectionsPortWindowSizeEnablesPortWindowMarginEnablesPortBufferSizeEnablesPortBufferMarginEnablesPortSynchronicityEnablesPortSignalSizeEnablesPortBufferSizesPortBufferMarginsFunctionDeclFunctionTemplateSpecKindFunctionTemplateParamNamesFunctionTemplateParamKindsFunctionTemplateParamTypesFunctionTemplateParamValuesFunctionTemplateParamEnablesClassDeclClassTemplateSpecKindClassTemplateParamNamesClassTemplateParamKindsClassTemplateParamTypesClassTemplateParamValuesClassTemplateParamEnablesClassCtorDeclsClassCtorParamNamesClassCtorParamTypesClassCtorParamSerializedTypes[1 1]@C[32 1]@t14@exp_calc_fixedt22@../../exp_calc_fixed.hC[2 1]@t9@cb_input1t10@cb_output1C[2 1]@t38@adf::input_buffer< cint16 > & restrictt39@adf::output_buffer< cint16 > & restrictC[2 1]@t42@{Q2{R{Tadf::input_buffer{1{t{Scint16}}}}}}t43@{Q2{R{Tadf::output_buffer{1{t{Scint16}}}}}}C[2 1]@t5@inputt6@outputC[2 1]@l1@l1@C[2 1]@l1@l0@C[2 1]@l1@l1@C[2 1]@l0@l0@C[2 1]@l1@l1@C[2 1]@l0@l0@C[2 1]@nnC[2 1]@nnt160@template < unsigned int PHASE_INDEX > 
      | void exp_calc_fixed(adf::input_buffer< cint16 > & restrict cb_input1, adf::output_buffer< cint16 > & restrict cb_output1)t8@implicitC[1 1]@t11@PHASE_INDEXC[1 1]@t7@nontypeC[1 1]@t12@unsigned intC[1 1]@nC[1 1]@l1@nne[0 1]@e[0 1]@e[0 1]@e[0 1]@e[0 1]@e[0 1]@e[0 1]@e[0 1]@e[0 1]@
      FunctionDeclTypeOptions=|
      | C[1 1]@t162@template < unsigned int PHASE_INDEX > 
      | void exp_calc_fixed(adf::input_buffer< cint16 > && restrict cb_input1, adf::output_buffer< cint16 > && restrict cb_output1)
      FunctionDecl=|
      | template < unsigned int PHASE_INDEX > 
      | void exp_calc_fixed(adf::input_buffer< cint16 > && restrict cb_input1, adf::output_buffer< cint16 > && restrict cb_output1)
  exp_calc_lookup_fixed_win6 : aieBasic/AIE Kernel  KernelAllAttrs=|  PortNames={'cb_input1'; 'cb_output1'}  PortSerializedTypes={'{Q2{R{Tadf::input_buffer{1{t{Scint16}}}}}}'; '{Q2{R{Tadf::output_buffer{1{t{Scint16}}}}}}'}  PortWindowSizes={2.048000000000000000e+03, 2.048000000000000000e+03}  PortWindowMargins={0.000000000000000000e+00, 0.000000000000000000e+00}  PortSynchronicities={'sync', 'sync'}  PortSignalSizes={0.000000000000000000e+00; 0.000000000000000000e+00}  FunctionTemplateSpecKind=implicit  FunctionTemplateParamNames={'PHASE_INDEX'}  FunctionTemplateParamKinds={'nontype'}  FunctionTemplateParamTypes={'unsigned int'}  FunctionTemplateParamValues={'6'}  FunctionIndex=1  FunctionTabVisible=on  FunctionTemplateParamsVisible=on  FunctionDeclTypeOptions=|  FunctionDecl=|  FunctionTemplateParams={ 'PHASE_INDEX', 'unsigned int', '6' }  FunctionTemplateParamsEnables={'off', 'off', 'on'}  PortAttrs={ 'input', 'cb_input1', 'adf::input_buffer< cint16 > & restrict', '2048', '0', 'sync', ''; 'output', 'cb_output1', 'adf::output_buffer< cint16 > & restrict', '2048', '', 'sync', '' }  PortAttrsEnables={'off', 'off', 'off', 'on', 'off', 'off', 'off';'off', 'off', 'off', 'on', 'off', 'off', 'off'}  SampleTime=-1  KernelHeaderFile=exp_calc_fixed.h  KernelFunction=exp_calc_fixed  KernelSourceFile=exp_calc_fixed.cc  KernelSearchPaths={}  PreProcOptions={}  blockJsonConstraints="{\"type\":\"constraint\",\"constraintType\":\"coreUtilization\",\"sid\":\"3285\",\"lhs\":{\"type\":\"runtimeRatio\",\"args\":{\"type\":\"kernel\",\"name\":\"fft32kpt_int_xpose/AIE_2kFFT_cplxRot/exp_calc_lookup_fixed_win6\",\"sid\":\"3285\"}},\"rhs\":{\"type\":\"evaluable\",\"expr\":\"0.2\",\"value\":0.2},\"equality\":true}"
      KernelAllAttrs=|
      | s[12;12;9;9;19;14;21;23;21;23;24;21;15;17;12;24;26;26;26;27;28;9;21;23;23;23;24;25;14;19;19;29]@FunctionNameDeclFileNamePortNamesPortTypesPortSerializedTypesPortDirectionsPortWindowSizeEnablesPortWindowMarginEnablesPortBufferSizeEnablesPortBufferMarginEnablesPortSynchronicityEnablesPortSignalSizeEnablesPortBufferSizesPortBufferMarginsFunctionDeclFunctionTemplateSpecKindFunctionTemplateParamNamesFunctionTemplateParamKindsFunctionTemplateParamTypesFunctionTemplateParamValuesFunctionTemplateParamEnablesClassDeclClassTemplateSpecKindClassTemplateParamNamesClassTemplateParamKindsClassTemplateParamTypesClassTemplateParamValuesClassTemplateParamEnablesClassCtorDeclsClassCtorParamNamesClassCtorParamTypesClassCtorParamSerializedTypes[1 1]@C[32 1]@t14@exp_calc_fixedt22@../../exp_calc_fixed.hC[2 1]@t9@cb_input1t10@cb_output1C[2 1]@t38@adf::input_buffer< cint16 > & restrictt39@adf::output_buffer< cint16 > & restrictC[2 1]@t42@{Q2{R{Tadf::input_buffer{1{t{Scint16}}}}}}t43@{Q2{R{Tadf::output_buffer{1{t{Scint16}}}}}}C[2 1]@t5@inputt6@outputC[2 1]@l1@l1@C[2 1]@l1@l0@C[2 1]@l1@l1@C[2 1]@l0@l0@C[2 1]@l1@l1@C[2 1]@l0@l0@C[2 1]@nnC[2 1]@nnt160@template < unsigned int PHASE_INDEX > 
      | void exp_calc_fixed(adf::input_buffer< cint16 > & restrict cb_input1, adf::output_buffer< cint16 > & restrict cb_output1)t8@implicitC[1 1]@t11@PHASE_INDEXC[1 1]@t7@nontypeC[1 1]@t12@unsigned intC[1 1]@nC[1 1]@l1@nne[0 1]@e[0 1]@e[0 1]@e[0 1]@e[0 1]@e[0 1]@e[0 1]@e[0 1]@e[0 1]@
      FunctionDeclTypeOptions=|
      | C[1 1]@t162@template < unsigned int PHASE_INDEX > 
      | void exp_calc_fixed(adf::input_buffer< cint16 > && restrict cb_input1, adf::output_buffer< cint16 > && restrict cb_output1)
      FunctionDecl=|
      | template < unsigned int PHASE_INDEX > 
      | void exp_calc_fixed(adf::input_buffer< cint16 > && restrict cb_input1, adf::output_buffer< cint16 > && restrict cb_output1)
  exp_calc_lookup_fixed_win7 : aieBasic/AIE Kernel  KernelAllAttrs=|  PortNames={'cb_input1'; 'cb_output1'}  PortSerializedTypes={'{Q2{R{Tadf::input_buffer{1{t{Scint16}}}}}}'; '{Q2{R{Tadf::output_buffer{1{t{Scint16}}}}}}'}  PortWindowSizes={2.048000000000000000e+03, 2.048000000000000000e+03}  PortWindowMargins={0.000000000000000000e+00, 0.000000000000000000e+00}  PortSynchronicities={'sync', 'sync'}  PortSignalSizes={0.000000000000000000e+00; 0.000000000000000000e+00}  FunctionTemplateSpecKind=implicit  FunctionTemplateParamNames={'PHASE_INDEX'}  FunctionTemplateParamKinds={'nontype'}  FunctionTemplateParamTypes={'unsigned int'}  FunctionTemplateParamValues={'7'}  FunctionIndex=1  FunctionTabVisible=on  FunctionTemplateParamsVisible=on  FunctionDeclTypeOptions=|  FunctionDecl=|  FunctionTemplateParams={ 'PHASE_INDEX', 'unsigned int', '7' }  FunctionTemplateParamsEnables={'off', 'off', 'on'}  PortAttrs={ 'input', 'cb_input1', 'adf::input_buffer< cint16 > & restrict', '2048', '0', 'sync', ''; 'output', 'cb_output1', 'adf::output_buffer< cint16 > & restrict', '2048', '', 'sync', '' }  PortAttrsEnables={'off', 'off', 'off', 'on', 'off', 'off', 'off';'off', 'off', 'off', 'on', 'off', 'off', 'off'}  SampleTime=-1  KernelHeaderFile=exp_calc_fixed.h  KernelFunction=exp_calc_fixed  KernelSourceFile=exp_calc_fixed.cc  KernelSearchPaths={}  PreProcOptions={}  blockJsonConstraints="{\"type\":\"constraint\",\"constraintType\":\"coreUtilization\",\"sid\":\"3286\",\"lhs\":{\"type\":\"runtimeRatio\",\"args\":{\"type\":\"kernel\",\"name\":\"fft32kpt_int_xpose/AIE_2kFFT_cplxRot/exp_calc_lookup_fixed_win7\",\"sid\":\"3286\"}},\"rhs\":{\"type\":\"evaluable\",\"expr\":\"0.2\",\"value\":0.2},\"equality\":true}"
      KernelAllAttrs=|
      | s[12;12;9;9;19;14;21;23;21;23;24;21;15;17;12;24;26;26;26;27;28;9;21;23;23;23;24;25;14;19;19;29]@FunctionNameDeclFileNamePortNamesPortTypesPortSerializedTypesPortDirectionsPortWindowSizeEnablesPortWindowMarginEnablesPortBufferSizeEnablesPortBufferMarginEnablesPortSynchronicityEnablesPortSignalSizeEnablesPortBufferSizesPortBufferMarginsFunctionDeclFunctionTemplateSpecKindFunctionTemplateParamNamesFunctionTemplateParamKindsFunctionTemplateParamTypesFunctionTemplateParamValuesFunctionTemplateParamEnablesClassDeclClassTemplateSpecKindClassTemplateParamNamesClassTemplateParamKindsClassTemplateParamTypesClassTemplateParamValuesClassTemplateParamEnablesClassCtorDeclsClassCtorParamNamesClassCtorParamTypesClassCtorParamSerializedTypes[1 1]@C[32 1]@t14@exp_calc_fixedt22@../../exp_calc_fixed.hC[2 1]@t9@cb_input1t10@cb_output1C[2 1]@t38@adf::input_buffer< cint16 > & restrictt39@adf::output_buffer< cint16 > & restrictC[2 1]@t42@{Q2{R{Tadf::input_buffer{1{t{Scint16}}}}}}t43@{Q2{R{Tadf::output_buffer{1{t{Scint16}}}}}}C[2 1]@t5@inputt6@outputC[2 1]@l1@l1@C[2 1]@l1@l0@C[2 1]@l1@l1@C[2 1]@l0@l0@C[2 1]@l1@l1@C[2 1]@l0@l0@C[2 1]@nnC[2 1]@nnt160@template < unsigned int PHASE_INDEX > 
      | void exp_calc_fixed(adf::input_buffer< cint16 > & restrict cb_input1, adf::output_buffer< cint16 > & restrict cb_output1)t8@implicitC[1 1]@t11@PHASE_INDEXC[1 1]@t7@nontypeC[1 1]@t12@unsigned intC[1 1]@nC[1 1]@l1@nne[0 1]@e[0 1]@e[0 1]@e[0 1]@e[0 1]@e[0 1]@e[0 1]@e[0 1]@e[0 1]@
      FunctionDeclTypeOptions=|
      | C[1 1]@t162@template < unsigned int PHASE_INDEX > 
      | void exp_calc_fixed(adf::input_buffer< cint16 > && restrict cb_input1, adf::output_buffer< cint16 > && restrict cb_output1)
      FunctionDecl=|
      | template < unsigned int PHASE_INDEX > 
      | void exp_calc_fixed(adf::input_buffer< cint16 > && restrict cb_input1, adf::output_buffer< cint16 > && restrict cb_output1)
  exp_calc_lookup_fixed_win8 : aieBasic/AIE Kernel  KernelAllAttrs=|  PortNames={'cb_input1'; 'cb_output1'}  PortSerializedTypes={'{Q2{R{Tadf::input_buffer{1{t{Scint16}}}}}}'; '{Q2{R{Tadf::output_buffer{1{t{Scint16}}}}}}'}  PortWindowSizes={2.048000000000000000e+03, 2.048000000000000000e+03}  PortWindowMargins={0.000000000000000000e+00, 0.000000000000000000e+00}  PortSynchronicities={'sync', 'sync'}  PortSignalSizes={0.000000000000000000e+00; 0.000000000000000000e+00}  FunctionTemplateSpecKind=implicit  FunctionTemplateParamNames={'PHASE_INDEX'}  FunctionTemplateParamKinds={'nontype'}  FunctionTemplateParamTypes={'unsigned int'}  FunctionTemplateParamValues={'8'}  FunctionIndex=1  FunctionTabVisible=on  FunctionTemplateParamsVisible=on  FunctionDeclTypeOptions=|  FunctionDecl=|  FunctionTemplateParams={ 'PHASE_INDEX', 'unsigned int', '8' }  FunctionTemplateParamsEnables={'off', 'off', 'on'}  PortAttrs={ 'input', 'cb_input1', 'adf::input_buffer< cint16 > & restrict', '2048', '0', 'sync', ''; 'output', 'cb_output1', 'adf::output_buffer< cint16 > & restrict', '2048', '', 'sync', '' }  PortAttrsEnables={'off', 'off', 'off', 'on', 'off', 'off', 'off';'off', 'off', 'off', 'on', 'off', 'off', 'off'}  SampleTime=-1  KernelHeaderFile=exp_calc_fixed.h  KernelFunction=exp_calc_fixed  KernelSourceFile=exp_calc_fixed.cc  KernelSearchPaths={}  PreProcOptions={}  blockJsonConstraints="{\"type\":\"constraint\",\"constraintType\":\"coreUtilization\",\"sid\":\"3287\",\"lhs\":{\"type\":\"runtimeRatio\",\"args\":{\"type\":\"kernel\",\"name\":\"fft32kpt_int_xpose/AIE_2kFFT_cplxRot/exp_calc_lookup_fixed_win8\",\"sid\":\"3287\"}},\"rhs\":{\"type\":\"evaluable\",\"expr\":\"0.2\",\"value\":0.2},\"equality\":true}"
      KernelAllAttrs=|
      | s[12;12;9;9;19;14;21;23;21;23;24;21;15;17;12;24;26;26;26;27;28;9;21;23;23;23;24;25;14;19;19;29]@FunctionNameDeclFileNamePortNamesPortTypesPortSerializedTypesPortDirectionsPortWindowSizeEnablesPortWindowMarginEnablesPortBufferSizeEnablesPortBufferMarginEnablesPortSynchronicityEnablesPortSignalSizeEnablesPortBufferSizesPortBufferMarginsFunctionDeclFunctionTemplateSpecKindFunctionTemplateParamNamesFunctionTemplateParamKindsFunctionTemplateParamTypesFunctionTemplateParamValuesFunctionTemplateParamEnablesClassDeclClassTemplateSpecKindClassTemplateParamNamesClassTemplateParamKindsClassTemplateParamTypesClassTemplateParamValuesClassTemplateParamEnablesClassCtorDeclsClassCtorParamNamesClassCtorParamTypesClassCtorParamSerializedTypes[1 1]@C[32 1]@t14@exp_calc_fixedt22@../../exp_calc_fixed.hC[2 1]@t9@cb_input1t10@cb_output1C[2 1]@t38@adf::input_buffer< cint16 > & restrictt39@adf::output_buffer< cint16 > & restrictC[2 1]@t42@{Q2{R{Tadf::input_buffer{1{t{Scint16}}}}}}t43@{Q2{R{Tadf::output_buffer{1{t{Scint16}}}}}}C[2 1]@t5@inputt6@outputC[2 1]@l1@l1@C[2 1]@l1@l0@C[2 1]@l1@l1@C[2 1]@l0@l0@C[2 1]@l1@l1@C[2 1]@l0@l0@C[2 1]@nnC[2 1]@nnt160@template < unsigned int PHASE_INDEX > 
      | void exp_calc_fixed(adf::input_buffer< cint16 > & restrict cb_input1, adf::output_buffer< cint16 > & restrict cb_output1)t8@implicitC[1 1]@t11@PHASE_INDEXC[1 1]@t7@nontypeC[1 1]@t12@unsigned intC[1 1]@nC[1 1]@l1@nne[0 1]@e[0 1]@e[0 1]@e[0 1]@e[0 1]@e[0 1]@e[0 1]@e[0 1]@e[0 1]@
      FunctionDeclTypeOptions=|
      | C[1 1]@t162@template < unsigned int PHASE_INDEX > 
      | void exp_calc_fixed(adf::input_buffer< cint16 > && restrict cb_input1, adf::output_buffer< cint16 > && restrict cb_output1)
      FunctionDecl=|
      | template < unsigned int PHASE_INDEX > 
      | void exp_calc_fixed(adf::input_buffer< cint16 > && restrict cb_input1, adf::output_buffer< cint16 > && restrict cb_output1)
  exp_calc_lookup_fixed_win9 : aieBasic/AIE Kernel  KernelAllAttrs=|  PortNames={'cb_input1'; 'cb_output1'}  PortSerializedTypes={'{Q2{R{Tadf::input_buffer{1{t{Scint16}}}}}}'; '{Q2{R{Tadf::output_buffer{1{t{Scint16}}}}}}'}  PortWindowSizes={2.048000000000000000e+03, 2.048000000000000000e+03}  PortWindowMargins={0.000000000000000000e+00, 0.000000000000000000e+00}  PortSynchronicities={'sync', 'sync'}  PortSignalSizes={0.000000000000000000e+00; 0.000000000000000000e+00}  FunctionTemplateSpecKind=implicit  FunctionTemplateParamNames={'PHASE_INDEX'}  FunctionTemplateParamKinds={'nontype'}  FunctionTemplateParamTypes={'unsigned int'}  FunctionTemplateParamValues={'9'}  FunctionIndex=1  FunctionTabVisible=on  FunctionTemplateParamsVisible=on  FunctionDeclTypeOptions=|  FunctionDecl=|  FunctionTemplateParams={ 'PHASE_INDEX', 'unsigned int', '9' }  FunctionTemplateParamsEnables={'off', 'off', 'on'}  PortAttrs={ 'input', 'cb_input1', 'adf::input_buffer< cint16 > & restrict', '2048', '0', 'sync', ''; 'output', 'cb_output1', 'adf::output_buffer< cint16 > & restrict', '2048', '', 'sync', '' }  PortAttrsEnables={'off', 'off', 'off', 'on', 'off', 'off', 'off';'off', 'off', 'off', 'on', 'off', 'off', 'off'}  SampleTime=-1  KernelHeaderFile=exp_calc_fixed.h  KernelFunction=exp_calc_fixed  KernelSourceFile=exp_calc_fixed.cc  KernelSearchPaths={}  PreProcOptions={}  blockJsonConstraints="{\"type\":\"constraint\",\"constraintType\":\"coreUtilization\",\"sid\":\"3288\",\"lhs\":{\"type\":\"runtimeRatio\",\"args\":{\"type\":\"kernel\",\"name\":\"fft32kpt_int_xpose/AIE_2kFFT_cplxRot/exp_calc_lookup_fixed_win9\",\"sid\":\"3288\"}},\"rhs\":{\"type\":\"evaluable\",\"expr\":\"0.2\",\"value\":0.2},\"equality\":true}"
      KernelAllAttrs=|
      | s[12;12;9;9;19;14;21;23;21;23;24;21;15;17;12;24;26;26;26;27;28;9;21;23;23;23;24;25;14;19;19;29]@FunctionNameDeclFileNamePortNamesPortTypesPortSerializedTypesPortDirectionsPortWindowSizeEnablesPortWindowMarginEnablesPortBufferSizeEnablesPortBufferMarginEnablesPortSynchronicityEnablesPortSignalSizeEnablesPortBufferSizesPortBufferMarginsFunctionDeclFunctionTemplateSpecKindFunctionTemplateParamNamesFunctionTemplateParamKindsFunctionTemplateParamTypesFunctionTemplateParamValuesFunctionTemplateParamEnablesClassDeclClassTemplateSpecKindClassTemplateParamNamesClassTemplateParamKindsClassTemplateParamTypesClassTemplateParamValuesClassTemplateParamEnablesClassCtorDeclsClassCtorParamNamesClassCtorParamTypesClassCtorParamSerializedTypes[1 1]@C[32 1]@t14@exp_calc_fixedt22@../../exp_calc_fixed.hC[2 1]@t9@cb_input1t10@cb_output1C[2 1]@t38@adf::input_buffer< cint16 > & restrictt39@adf::output_buffer< cint16 > & restrictC[2 1]@t42@{Q2{R{Tadf::input_buffer{1{t{Scint16}}}}}}t43@{Q2{R{Tadf::output_buffer{1{t{Scint16}}}}}}C[2 1]@t5@inputt6@outputC[2 1]@l1@l1@C[2 1]@l1@l0@C[2 1]@l1@l1@C[2 1]@l0@l0@C[2 1]@l1@l1@C[2 1]@l0@l0@C[2 1]@nnC[2 1]@nnt160@template < unsigned int PHASE_INDEX > 
      | void exp_calc_fixed(adf::input_buffer< cint16 > & restrict cb_input1, adf::output_buffer< cint16 > & restrict cb_output1)t8@implicitC[1 1]@t11@PHASE_INDEXC[1 1]@t7@nontypeC[1 1]@t12@unsigned intC[1 1]@nC[1 1]@l1@nne[0 1]@e[0 1]@e[0 1]@e[0 1]@e[0 1]@e[0 1]@e[0 1]@e[0 1]@e[0 1]@
      FunctionDeclTypeOptions=|
      | C[1 1]@t162@template < unsigned int PHASE_INDEX > 
      | void exp_calc_fixed(adf::input_buffer< cint16 > && restrict cb_input1, adf::output_buffer< cint16 > && restrict cb_output1)
      FunctionDecl=|
      | template < unsigned int PHASE_INDEX > 
      | void exp_calc_fixed(adf::input_buffer< cint16 > && restrict cb_input1, adf::output_buffer< cint16 > && restrict cb_output1)
  Out1 : Outport
  Out2 : Outport  Port=2
  Out3 : Outport  Port=3
  Out4 : Outport  Port=4
  Out5 : Outport  Port=5
  Out6 : Outport  Port=6
  Out7 : Outport  Port=7
  Out8 : Outport  Port=8
  Out9 : Outport  Port=9
  Out10 : Outport  Port=10
  Out11 : Outport  Port=11
  Out12 : Outport  Port=12
  Out13 : Outport  Port=13
  Out14 : Outport  Port=14
  Out15 : Outport  Port=15
  Out16 : Outport  Port=16
  wires:
  PLIO23/1 -> Out16/1
  exp_calc_lookup_fixed_win14/1 -> PLIO22/1
  In3/1 -> PLIO2/1
  exp_calc_lookup_fixed_win9/1 -> PLIO31/1
  PLIO17/1 -> Out2/1
  PLIO28/1 -> Out7/1
  exp_calc_lookup_fixed_win7/1 -> PLIO29/1
  PLIO27/1 -> Out6/1
  PLIO19/1 -> Out12/1
  In14/1 -> PLIO13/1
  PLIO26/1 -> Out5/1
  In8/1 -> PLIO7/1
  exp_calc_lookup_fixed_win5/1 -> PLIO27/1
  In4/1 -> PLIO3/1
  PLIO29/1 -> Out8/1
  In6/1 -> PLIO5/1
  exp_calc_lookup_fixed_win2/1 -> PLIO24/1
  PLIO25/1 -> Out4/1
  In7/1 -> PLIO6/1
  PLIO31/1 -> Out10/1
  In12/1 -> PLIO11/1
  PLIO30/1 -> Out9/1
  In2/1 -> PLIO1/1
  PLIO24/1 -> Out3/1
  exp_calc_lookup_fixed_win8/1 -> PLIO30/1
  exp_calc_lookup_fixed_win12/1 -> PLIO20/1
  PLIO21/1 -> Out14/1
  In15/1 -> PLIO14/1
  exp_calc_lookup_fixed_win4/1 -> PLIO26/1
  PLIO22/1 -> Out15/1
  In16/1 -> PLIO15/1
  PLIO16/1 -> Out1/1
  In11/1 -> PLIO10/1
  In5/1 -> PLIO4/1
  exp_calc_lookup_fixed_win11/1 -> PLIO19/1
  PLIO20/1 -> Out13/1
  In10/1 -> PLIO9/1
  exp_calc_lookup_fixed_win10/1 -> PLIO18/1
  exp_calc_lookup_fixed_win6/1 -> PLIO28/1
  PLIO18/1 -> Out11/1
  exp_calc_lookup_fixed_win15/1 -> PLIO23/1
  In13/1 -> PLIO12/1
  In9/1 -> PLIO8/1
  PLIO/1 -> FFT/1
  PLIO1/1 -> FFT1/1
  PLIO2/1 -> FFT2/1
  PLIO3/1 -> FFT3/1
  PLIO6/1 -> FFT6/1
  PLIO4/1 -> FFT4/1
  PLIO5/1 -> FFT5/1
  PLIO7/1 -> FFT7/1
  PLIO12/1 -> FFT12/1
  PLIO11/1 -> FFT11/1
  PLIO8/1 -> FFT8/1
  PLIO10/1 -> FFT10/1
  PLIO9/1 -> FFT9/1
  PLIO14/1 -> FFT14/1
  PLIO15/1 -> FFT15/1
  PLIO13/1 -> FFT13/1
  FFT/1 -> PLIO16/1
  FFT2/1 -> exp_calc_lookup_fixed_win2/1
  FFT5/1 -> exp_calc_lookup_fixed_win5/1
  FFT6/1 -> exp_calc_lookup_fixed_win6/1
  FFT7/1 -> exp_calc_lookup_fixed_win7/1
  FFT4/1 -> exp_calc_lookup_fixed_win4/1
  FFT8/1 -> exp_calc_lookup_fixed_win8/1
  FFT14/1 -> exp_calc_lookup_fixed_win14/1
  FFT10/1 -> exp_calc_lookup_fixed_win10/1
  FFT11/1 -> exp_calc_lookup_fixed_win11/1
  FFT13/1 -> exp_calc_lookup_fixed_win13/1
  FFT15/1 -> exp_calc_lookup_fixed_win15/1
  FFT12/1 -> exp_calc_lookup_fixed_win12/1
  FFT9/1 -> exp_calc_lookup_fixed_win9/1
  In1/1 -> PLIO/1
  exp_calc_lookup_fixed_win13/1 -> PLIO21/1
  FFT1/1 -> exp_calc_fixed/1
  exp_calc_fixed/1 -> PLIO17/1
  FFT3/1 -> exp_calc_fixed1/1
  exp_calc_fixed1/1 -> PLIO25/1
